simulink model "PD_rigid"  (R2021b)
settings: Solver=VariableStepAuto  StartTime=0.0  StopTime=10.0  RelTol=1e-3
undefined symbols (not defined in the file): Kd, Kp, qd
settings Model: Creator=fabioscap  LastModifiedBy=fabioscap

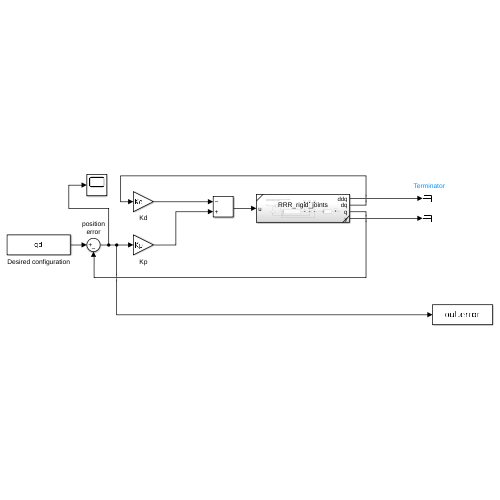
[thumbnail: Simulink's stored preview of the top-level diagram]
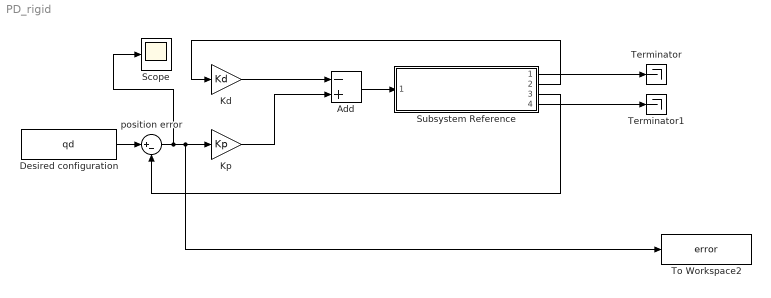
== system PD_rigid ==
  Add : Sum  Inputs=-+
  Desired configuration : Constant  Value=qd
  Kd : Gain  Gain=Kd
  Kp : Gain  Gain=Kp
  Scope : Scope
  Subsystem Reference : Subsystem  ReferencedSubsystem=RRR_rigid_joints
  Terminator : Terminator
  Terminator1 : Terminator
  To Workspace2 : ToWorkspace  VariableName=error  SaveFormat=Timeseries  SampleTime=-1
  position error : Sum  Inputs=|+-
  wires:
  Add/1 -> Subsystem Reference/1
  Kd/1 -> Add/1
  Kp/1 -> Add/2
  Subsystem Reference/2 -> Kd/1
  Subsystem Reference/3 -> position error/2
  Desired configuration/1 -> position error/1
  position error/1 -> Scope/1, To Workspace2/1, Kp/1
  Subsystem Reference/1 -> Terminator/1
  Subsystem Reference/4 -> Terminator1/1
